simulink model "model"  (R2022a)
settings: Solver=VariableStepAuto  StartTime=0.0  StopTime=20  RelTol=1e-3
values from neighbouring files (symbols this model uses):
  b_0 = 7    [config.m]
  gamma = 10000    [config.m]    (also in task_kras.m = 10000000000; tasks.m = 100000000; test_grad.m = 1000)
  k_0 = 1    [config.m]
  K_M = K_M_g    [config.m]
  nu1 = zeros(length(Lambda), 1)    [config.m]
  nu2 = zeros(length(Lambda), 1)    [config.m]
  object_denum = [1 a_1 a_0]    [config.m]
  object_num = [b_0]    [config.m]
  psi_hat_init_conds = zeros(omega_size, 1)    [config.m]
settings Model: LastModifiedBy=Vvlad
settings OptimizationCC: BlockReduction=off  BooleanDataType=off
settings DebuggingCC: SaveWithParameterizedLinksMsg=none  UnderspecifiedInitializationDetection=Classic  MergeDetectMultiDrivingBlocksExec=none  SignalResolutionControl=TryResolveAllWithWarning  UnconnectedInputMsg=warning  UnconnectedOutputMsg=warning  UnconnectedLineMsg=warning
settings HardwareCC: TargetUnknown=on
settings ModelReferenceCC: PropagateSignalLabelsOutOfModel=off
settings RTWCC: DLArmComputeVersion=19.05

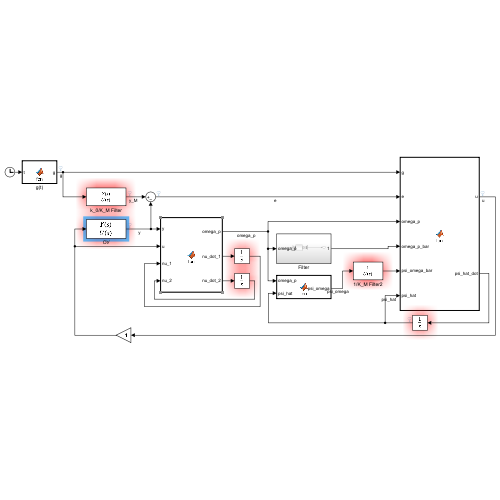
[thumbnail: Simulink's stored preview of the top-level diagram]
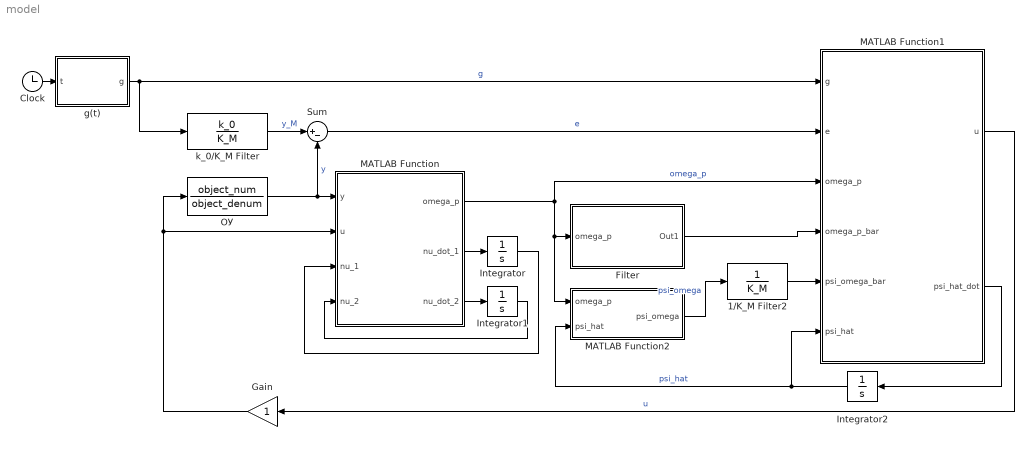
== system model ==
  1/K_M Filter2 : TransferFcn  Denominator=K_M
  Clock : Clock
  Filter : Subsystem
  Gain : Gain
  Integrator : Integrator  InitialCondition=nu1
  Integrator1 : Integrator  InitialCondition=nu2
  Integrator2 : Integrator  InitialCondition=psi_hat_init_conds
  MATLAB Function : MATLAB Function  TreatAsAtomicUnit=on
  MATLAB Function1 : MATLAB Function  TreatAsAtomicUnit=on
  MATLAB Function2 : MATLAB Function  TreatAsAtomicUnit=on
  Sum : Sum  Inputs=|+-
  g(t) : MATLAB Function  TreatAsAtomicUnit=on
  k_0/K_M Filter : TransferFcn  Numerator=k_0  Denominator=K_M
  ОУ : TransferFcn  Numerator=object_num  Denominator=object_denum
  wires:
  MATLAB Function/3(nu_dot_2) -> Integrator1/1
  MATLAB Function/2(nu_dot_1) -> Integrator/1
  Integrator1/1 -> MATLAB Function/4(nu_2)
  Integrator/1 -> MATLAB Function/3(nu_1)
  ОУ/1 -> MATLAB Function/1(y), Sum/2  "y"
  MATLAB Function1/1(u) -> Gain/1  "u"
  Clock/1 -> g(t)/1(t)
  g(t)/1(g) -> k_0/K_M Filter/1, MATLAB Function1/1(g)  "g"
  k_0/K_M Filter/1 -> Sum/1  "y_M"
  Sum/1 -> MATLAB Function1/2(e)  "e"
  MATLAB Function/1(omega_p) -> MATLAB Function1/3(omega_p), Filter/1(omega_p), MATLAB Function2/1(omega_p)  "omega_p"
  MATLAB Function1/2(psi_hat_dot) -> Integrator2/1
  Integrator2/1 -> MATLAB Function2/2(psi_hat), MATLAB Function1/6(psi_hat)  "psi_hat"
  1/K_M Filter2/1 -> MATLAB Function1/5(psi_omega_bar)
  MATLAB Function2/1(psi_omega) -> 1/K_M Filter2/1  "psi_omega"
  Gain/1 -> MATLAB Function/2(u), ОУ/1
  Filter/1(Out1) -> MATLAB Function1/4(omega_p_bar)

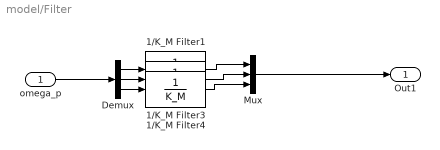
== system model/Filter ==
  omega_p : Inport
  1/K_M Filter1 : TransferFcn  Denominator=K_M
  1/K_M Filter3 : TransferFcn  Denominator=K_M
  1/K_M Filter4 : TransferFcn  Denominator=K_M
  Demux : Demux  Outputs=3
  Mux : Mux  Inputs=3
  Out1 : Outport
  wires:
  1/K_M Filter1/1 -> Mux/1
  Demux/2 -> 1/K_M Filter3/1
  Demux/3 -> 1/K_M Filter4/1
  1/K_M Filter4/1 -> Mux/3
  Mux/1 -> Out1/1
  1/K_M Filter3/1 -> Mux/2
  Demux/1 -> 1/K_M Filter1/1
  omega_p/1 -> Demux/1

== matlab function model/MATLAB Function ==
  data: y input; u input; omega_p output; nu_1 input; nu_2 input; nu_dot_1 output; nu_dot_2 output; Lambda parameter
function [omega_p, nu_dot_1, nu_dot_2] = fcn(y, u, nu_1, nu_2, Lambda)

nu_dot_1 = Lambda*nu_1 + u;
nu_dot_2 = Lambda*nu_2 + y;
omega = [nu_1', nu_2', y]';
omega_p = -omega;

== matlab function model/g(t) ==
  data: t input; g output
function g = fcn(t)

g = 7*sin(8*t+1);

== matlab function model/MATLAB Function1 ==
  data: g input; e input; u output; omega_p input; omega_p_bar input; psi_hat_dot output; psi_omega_bar input; gamma parameter; k_0 parameter; b_0 parameter; psi_hat input
function [u,psi_hat_dot] = fcn(g,e,omega_p,omega_p_bar, psi_omega_bar, gamma, k_0, b_0, psi_hat)

e_hat = e - psi_hat'*omega_p_bar + psi_omega_bar;
psi_hat_dot = gamma*omega_p_bar*e_hat/(1+omega_p_bar'*omega_p_bar);
u = (psi_hat'*omega_p+k_0*g)/b_0;

== matlab function model/MATLAB Function2 ==
  data: omega_p input; psi_hat input; psi_omega output
function psi_omega = fcn(omega_p, psi_hat)
 psi_omega = psi_hat'*omega_p;
